simulink model "OFDM_Tx_HW"  (R2020a)
settings: Solver=FixedStepDiscrete  StartTime=0.0  StopTime=inf  RelTol=1e-3
InitFcn:
  | % Set parameters
  | fs = 1e6;
  | 
  | % Load all required variables
  | load('variables/read_addr_data');
  | load('variables/read_addr_cp');
  | load('variables/read_addr_pream');
  | load('variables/read_addr_rx');
  | load('variables/pilot');
  | load('variables/sc_index');
  | load('variables/LTSfreq');
  | load('variables/STSfreq');
  | load('variables/LTSread');
  | load('variables/STSread');
  | 
  | run ./scripts/rfgen;
undefined symbols (not defined in the file or in its folder): CIC_fine_Rx, LTSfreq, LTSread, pilot, read_addr_cp, read_addr_data, read_addr_pream, STSfreq, STSread
libraries: hdlsllib x47, xbsIndex_r4 x30, simulink x19, xrbsSSR_Library x8, dspsigops x5, dspmlti4 x3, lib_ofdmrx x1, lib_rfsignalgenerator x1, dsphdlxfrm x1, dspobslib x1
(part 2 of 2)

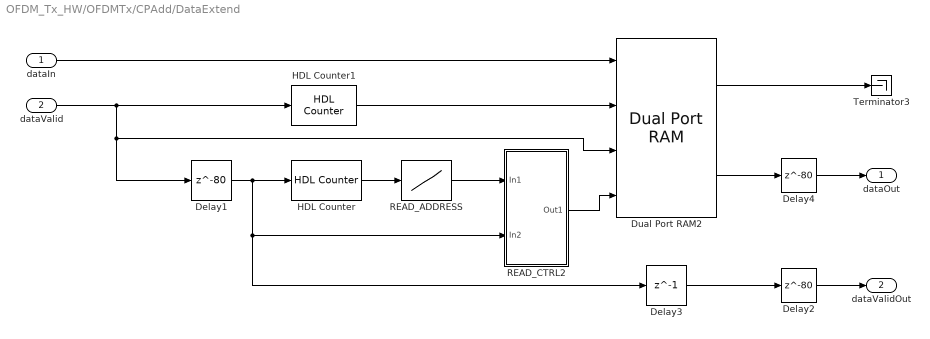
== system OFDM_Tx_HW/OFDMTx/CPAdd/DataExtend ==
  dataIn : Inport
  dataValid : Inport  Port=2
  Delay1 : Delay  DelayLength=80  InitialCondition=0  UseCircularBuffer=on
  Delay2 : Delay  DelayLength=80
  Delay3 : Delay  DelayLength=1  InitialCondition=0  UseCircularBuffer=on
  Delay4 : Delay  DelayLength=80
  Dual Port RAM2 : hdlsllib/HDL RAMs/Dual Port RAM  ram_size=8
      settings: SourceProductBaseCode=SL
  HDL Counter : hdlsllib/Sources/HDL Counter  CountType=Count limited  CountInit=0  CountStep=1  CountMax=159  CountFromType=Initial value  CountFrom=0  CountResetPort=off  CountLoadPort=off  CountEnbPort=on  CountDirPort=off  CountDataType=Unsigned  CountWordLen=8  CountFracLen=0  CountSampTime=1
  HDL Counter1 : hdlsllib/Sources/HDL Counter  CountType=Count limited  CountInit=0  CountStep=1  CountMax=159  CountFromType=Initial value  CountFrom=0  CountResetPort=off  CountLoadPort=off  CountEnbPort=on  CountDirPort=off  CountDataType=Unsigned  CountWordLen=8  CountFracLen=0  CountSampTime=1
  READ_ADDRESS : Lookup_n-D  NumberOfTableDimensions=1  LookupTableObject=''  BreakpointsForDimension1=[0:159]  BreakpointsForDimension1FirstPoint=10  BreakpointsForDimension2FirstPoint=10  BreakpointsForDimension1Spacing=12  BreakpointsForDimension2Spacing=12  IndexSearchMethod=Evenly spaced points  Table=read_addr_cp  TableDataTypeStr=fixdt(0,8,0)  InterpMethod=Flat  DiagnosticForOutOfRangeInput=Error  InternalRulePriority=Speed  OutDataTypeStr=fixdt(0,8,0)  RndMeth=Simplest  InputSameDT=on
  READ_CTRL2 : Subsystem
  Terminator3 : Terminator
  dataOut : Outport  VectorParamsAs1DForOutWhenUnconnected=off
  dataValidOut : Outport  Port=2  VectorParamsAs1DForOutWhenUnconnected=off
  wires:
  Delay4/1 -> dataOut/1
  Delay2/1 -> dataValidOut/1
  Dual Port RAM2/1 -> Terminator3/1
  READ_ADDRESS/1 -> READ_CTRL2/1(In1)
  HDL Counter/1 -> READ_ADDRESS/1
  dataIn/1 -> Dual Port RAM2/1
  HDL Counter1/1 -> Dual Port RAM2/2
  Delay1/1 -> HDL Counter/1, Delay3/1, READ_CTRL2/2(In2)
  Dual Port RAM2/2 -> Delay4/1
  dataValid/1 -> HDL Counter1/1, Dual Port RAM2/3, Delay1/1
  Delay3/1 -> Delay2/1
  READ_CTRL2/1(Out1) -> Dual Port RAM2/4

== system OFDM_Tx_HW/OFDMTx/CPAdd/LTFExtend ==
  data : Inport
  preambVal : Inport  Port=2
  Delay : Delay  DelayLength=160  InitialCondition=0  UseCircularBuffer=on
  Delay12 : Delay  DelayLength=1  InitialCondition=0  UseCircularBuffer=on
  Dual Port RAM : hdlsllib/HDL RAMs/Dual Port RAM  ram_size=8
      settings: SourceProductBaseCode=SL
  HDL Counter2 : hdlsllib/Sources/HDL Counter  CountType=Count limited  CountInit=0  CountStep=1  CountMax=159  CountFromType=Initial value  CountFrom=0  CountResetPort=off  CountLoadPort=off  CountEnbPort=on  CountDirPort=off  CountDataType=Unsigned  CountWordLen=8  CountFracLen=0  CountSampTime=1
  HDL Counter3 : hdlsllib/Sources/HDL Counter  CountType=Count limited  CountInit=0  CountStep=1  CountMax=159  CountFromType=Initial value  CountFrom=0  CountResetPort=off  CountLoadPort=off  CountEnbPort=on  CountDirPort=off  CountDataType=Unsigned  CountWordLen=8  CountFracLen=0  CountSampTime=1
  LTFValidGen : Subsystem
  READ_CTRL : Subsystem
  Terminator1 : Terminator
  readaddr : Lookup_n-D  NumberOfTableDimensions=1  LookupTableObject=''  BreakpointsForDimension1=0:159  BreakpointsForDimension1FirstPoint=10  BreakpointsForDimension2FirstPoint=10  BreakpointsForDimension1Spacing=12  BreakpointsForDimension2Spacing=12  IndexSearchMethod=Evenly spaced points  Table=LTSread  TableDataTypeStr=fixdt(0,8,0)  InterpMethod=Flat  DiagnosticForOutOfRangeInput=Error  InternalRulePriority=Speed  OutDataTypeStr=fixdt(0,8,0)  RndMeth=Simplest  InputSameDT=on
  LTFExtendOut : Outport  VectorParamsAs1DForOutWhenUnconnected=off
  LTFValidOut : Outport  Port=2  VectorParamsAs1DForOutWhenUnconnected=off
  wires:
  readaddr/1 -> READ_CTRL/1(In1)
  READ_CTRL/1(Out1) -> Dual Port RAM/4
  HDL Counter3/1 -> Dual Port RAM/2
  Delay/1 -> READ_CTRL/2(In2), Delay12/1, HDL Counter2/1
  Dual Port RAM/1 -> Terminator1/1
  Delay12/1 -> LTFValidOut/1
  HDL Counter2/1 -> readaddr/1
  data/1 -> Dual Port RAM/1
  Dual Port RAM/2 -> LTFExtendOut/1
  preambVal/1 -> LTFValidGen/1(In1)
  LTFValidGen/1(Out1) -> Dual Port RAM/3, Delay/1, HDL Counter3/1

== system OFDM_Tx_HW/OFDMTx/CPAdd/STFExtend ==
  data : Inport
  preambVal : Inport  Port=2
  Delay : Delay  DelayLength=160  InitialCondition=0  UseCircularBuffer=on
  Delay12 : Delay  DelayLength=1  InitialCondition=0  UseCircularBuffer=on
  Dual Port RAM : hdlsllib/HDL RAMs/Dual Port RAM  ram_size=8
      settings: SourceProductBaseCode=SL
  HDL Counter2 : hdlsllib/Sources/HDL Counter  CountType=Count limited  CountInit=0  CountStep=1  CountMax=159  CountFromType=Initial value  CountFrom=0  CountResetPort=off  CountLoadPort=off  CountEnbPort=on  CountDirPort=off  CountDataType=Unsigned  CountWordLen=8  CountFracLen=0  CountSampTime=1
  HDL Counter3 : hdlsllib/Sources/HDL Counter  CountType=Count limited  CountInit=0  CountStep=1  CountMax=159  CountFromType=Initial value  CountFrom=0  CountResetPort=off  CountLoadPort=off  CountEnbPort=on  CountDirPort=off  CountDataType=Unsigned  CountWordLen=8  CountFracLen=0  CountSampTime=1
  READ_CTRL : Subsystem
  STFValidGen : Subsystem
  Terminator1 : Terminator
  readaddr : Lookup_n-D  NumberOfTableDimensions=1  LookupTableObject=''  BreakpointsForDimension1=0:159  BreakpointsForDimension1FirstPoint=10  BreakpointsForDimension2FirstPoint=10  BreakpointsForDimension1Spacing=12  BreakpointsForDimension2Spacing=12  IndexSearchMethod=Evenly spaced points  Table=STSread  TableDataTypeStr=fixdt(0,8,0)  InterpMethod=Flat  DiagnosticForOutOfRangeInput=Error  InternalRulePriority=Speed  OutDataTypeStr=fixdt(0,8,0)  RndMeth=Simplest  InputSameDT=on
  STFExtendOut : Outport  VectorParamsAs1DForOutWhenUnconnected=off
  STFValidOut : Outport  Port=2  VectorParamsAs1DForOutWhenUnconnected=off
  wires:
  Dual Port RAM/2 -> STFExtendOut/1
  data/1 -> Dual Port RAM/1
  HDL Counter2/1 -> readaddr/1
  Delay12/1 -> STFValidOut/1
  Dual Port RAM/1 -> Terminator1/1
  Delay/1 -> HDL Counter2/1, Delay12/1, READ_CTRL/2(In2)
  HDL Counter3/1 -> Dual Port RAM/2
  READ_CTRL/1(Out1) -> Dual Port RAM/4
  preambVal/1 -> STFValidGen/1(In1)
  readaddr/1 -> READ_CTRL/1(In1)
  STFValidGen/1(Out1) -> HDL Counter3/1, Dual Port RAM/3, Delay/1

== system OFDM_Tx_HW/OFDMTx/ControlSignalGenerator/PreamValidGen ==
  enable : Inport
  Compare To Constant : simulink/Logic and Bit Operations/Compare To Constant  relop===  const=320  OutDataTypeStr=boolean
  HDL Counter : hdlsllib/Sources/HDL Counter  CountType=Count limited  CountInit=0  CountStep=1  CountMax=320  CountFromType=Initial value  CountFrom=0  CountResetPort=on  CountLoadPort=off  CountEnbPort=on  CountDirPort=off  CountDataType=Unsigned  CountWordLen=9  CountFracLen=0  CountSampTime=1
  NOT : Logic  Operator=NOT  IconShape=distinctive  AllPortsSameDT=off  OutDataTypeStr=boolean
  RisingEdge : Subsystem
  Unit Delay Enabled Resettable Synchronous : hdlsllib/Discrete/Unit Delay Enabled Resettable Synchronous  InitialCondition=0.0  SampleTime=-1
      settings: SourceProductBaseCode=SL
  y : Outport  VectorParamsAs1DForOutWhenUnconnected=off
  wires:
  HDL Counter/1 -> Compare To Constant/1
  RisingEdge/1(Out1) -> Unit Delay Enabled Resettable Synchronous/2
  Compare To Constant/1 -> Unit Delay Enabled Resettable Synchronous/3
  enable/1 -> RisingEdge/1(In1), Unit Delay Enabled Resettable Synchronous/1, NOT/1, HDL Counter/2
  Unit Delay Enabled Resettable Synchronous/1 -> y/1
  NOT/1 -> HDL Counter/1

== system OFDM_Tx_HW/OFDMTx/ControlSignalGenerator/dataReadyGen ==
  enb : Inport
  Compare To Constant : simulink/Logic and Bit Operations/Compare To Constant  relop=>  const=31  OutDataTypeStr=boolean
  HDL Counter : hdlsllib/Sources/HDL Counter  CountType=Count limited  CountInit=0  CountStep=1  CountMax=79  CountFromType=Initial value  CountFrom=0  CountResetPort=on  CountLoadPort=off  CountEnbPort=on  CountDirPort=off  CountDataType=Unsigned  CountWordLen=7  CountFracLen=0  CountSampTime=1
  NOT : Logic  Operator=NOT  IconShape=distinctive  AllPortsSameDT=off  OutDataTypeStr=boolean
  y : Outport
  wires:
  HDL Counter/1 -> Compare To Constant/1
  enb/1 -> NOT/1, HDL Counter/2
  NOT/1 -> HDL Counter/1
  Compare To Constant/1 -> y/1

== system OFDM_Tx_HW/OFDMTx/ControlSignalGenerator/dataValidGen ==
  y : Inport
  enable : Inport  Port=2
  AND : Logic  IconShape=distinctive  AllPortsSameDT=off  OutDataTypeStr=boolean
  Delay : Delay  DelayLength=1
  NOT : Logic  Operator=NOT  IconShape=distinctive  AllPortsSameDT=off  OutDataTypeStr=boolean
  valOut : Outport
  wires:
  NOT/1 -> AND/1
  Delay/1 -> AND/2
  AND/1 -> valOut/1
  y/1 -> NOT/1
  enable/1 -> Delay/1

== system OFDM_Tx_HW/OFDMTx/ControlSignalGenerator/pilotValidGen ==
  enb : Inport
  AND : Logic  IconShape=distinctive  AllPortsSameDT=off  OutDataTypeStr=boolean
  Compare To Constant : simulink/Logic and Bit Operations/Compare To Constant  relop=<  const=32  OutDataTypeStr=boolean
  Compare To Constant1 : simulink/Logic and Bit Operations/Compare To Constant  relop=>  const=27  OutDataTypeStr=boolean
  HDL Counter : hdlsllib/Sources/HDL Counter  CountType=Count limited  CountInit=0  CountStep=1  CountMax=79  CountFromType=Initial value  CountFrom=0  CountResetPort=on  CountLoadPort=off  CountEnbPort=on  CountDirPort=off  CountDataType=Unsigned  CountWordLen=7  CountFracLen=0  CountSampTime=1
  NOT : Logic  Operator=NOT  IconShape=distinctive  AllPortsSameDT=off  OutDataTypeStr=boolean
  y : Outport
  wires:
  NOT/1 -> HDL Counter/1
  enb/1 -> HDL Counter/2, NOT/1
  HDL Counter/1 -> Compare To Constant1/1, Compare To Constant/1
  Compare To Constant/1 -> AND/1
  Compare To Constant1/1 -> AND/2
  AND/1 -> y/1

== system OFDM_Tx_HW/OFDMTx/DataGenerator/LTSfreq ==
  preambVal : Inport
  AND : Logic  IconShape=distinctive  AllPortsSameDT=off  OutDataTypeStr=boolean
  AND1 : Logic  IconShape=distinctive  AllPortsSameDT=off  OutDataTypeStr=boolean
  Compare To Constant : simulink/Logic and Bit Operations/Compare To Constant  relop=>=  const=256  OutDataTypeStr=boolean
  Compare To Constant1 : simulink/Logic and Bit Operations/Compare To Constant  relop=<=  const=319  OutDataTypeStr=boolean
  HDL Counter1 : hdlsllib/Sources/HDL Counter  CountType=Count limited  CountInit=0  CountStep=1  CountMax=319  CountFromType=Initial value  CountFrom=0  CountResetPort=on  CountLoadPort=off  CountEnbPort=on  CountDirPort=off  CountDataType=Unsigned  CountWordLen=9  CountFracLen=0  CountSampTime=1
  HDL Counter4 : hdlsllib/Sources/HDL Counter  CountType=Count limited  CountInit=0  CountStep=1  CountMax=63  CountFromType=Initial value  CountFrom=0  CountResetPort=off  CountLoadPort=off  CountEnbPort=on  CountDirPort=off  CountDataType=Unsigned  CountWordLen=6  CountFracLen=0  CountSampTime=1
  LTSFreq : Lookup_n-D  NumberOfTableDimensions=1  LookupTableObject=''  BreakpointsForDimension1=0:63  BreakpointsForDimension1FirstPoint=10  BreakpointsForDimension2FirstPoint=10  BreakpointsForDimension1Spacing=12  BreakpointsForDimension2Spacing=12  IndexSearchMethod=Evenly spaced points  Table=LTSfreq  TableDataTypeStr=fixdt(1,16,14)  InterpMethod=Flat  DiagnosticForOutOfRangeInput=Error  InternalRulePriority=Speed  OutDataTypeStr=fixdt(1,16,14)  RndMeth=Simplest  InputSameDT=on
  NOT : Logic  Operator=NOT  IconShape=distinctive  AllPortsSameDT=off  OutDataTypeStr=boolean
  ltsFreq : Outport  VectorParamsAs1DForOutWhenUnconnected=off
  ltsVal : Outport  Port=2  VectorParamsAs1DForOutWhenUnconnected=off
  wires:
  HDL Counter4/1 -> LTSFreq/1
  Compare To Constant/1 -> AND/1
  HDL Counter1/1 -> Compare To Constant1/1, Compare To Constant/1
  Compare To Constant1/1 -> AND/2
  NOT/1 -> HDL Counter1/1
  AND/1 -> AND1/1
  preambVal/1 -> NOT/1, AND1/2, HDL Counter1/2
  AND1/1 -> ltsVal/1, HDL Counter4/1
  LTSFreq/1 -> ltsFreq/1

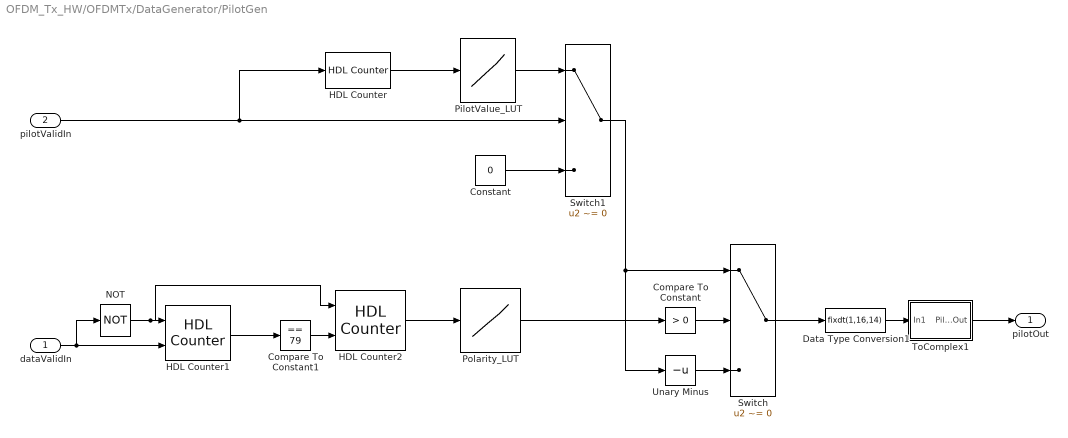
== system OFDM_Tx_HW/OFDMTx/DataGenerator/PilotGen ==
  dataValidIn : Inport
  pilotValidIn : Inport  Port=2
  Compare To Constant : simulink/Logic and Bit Operations/Compare To Constant  relop=>  const=0  OutDataTypeStr=boolean
  Compare To Constant1 : simulink/Logic and Bit Operations/Compare To Constant  relop===  const=79  OutDataTypeStr=boolean
  Constant : Constant  Value=0  OutDataTypeStr=fixdt(1,2,0)  SampleTime=1/fs
  Data Type Conversion1 : DataTypeConversion  OutDataTypeStr=fixdt(1,16,14)
  HDL Counter : hdlsllib/Sources/HDL Counter  CountType=Count limited  CountInit=0  CountStep=1  CountMax=3  CountFromType=Initial value  CountFrom=0  CountResetPort=off  CountLoadPort=off  CountEnbPort=on  CountDirPort=off  CountDataType=Unsigned  CountWordLen=2  CountFracLen=0  CountSampTime=1
  HDL Counter1 : hdlsllib/Sources/HDL Counter  CountType=Count limited  CountInit=0  CountStep=1  CountMax=79  CountFromType=Initial value  CountFrom=0  CountResetPort=on  CountLoadPort=off  CountEnbPort=on  CountDirPort=off  CountDataType=Unsigned  CountWordLen=8  CountFracLen=0  CountSampTime=1
  HDL Counter2 : hdlsllib/Sources/HDL Counter  CountType=Count limited  CountInit=0  CountStep=1  CountMax=126  CountFromType=Initial value  CountFrom=0  CountResetPort=on  CountLoadPort=off  CountEnbPort=on  CountDirPort=off  CountDataType=Unsigned  CountWordLen=7  CountFracLen=0  CountSampTime=1
  NOT : Logic  Operator=NOT  IconShape=distinctive  AllPortsSameDT=off  OutDataTypeStr=boolean
  PilotValue_LUT : Lookup_n-D  NumberOfTableDimensions=1  LookupTableObject=''  BreakpointsForDimension1=[0:3]  BreakpointsForDimension1FirstPoint=10  BreakpointsForDimension2FirstPoint=10  BreakpointsForDimension1Spacing=12  BreakpointsForDimension2Spacing=12  IndexSearchMethod=Evenly spaced points  Table=[1 1 1 -1]  TableDataTypeStr=fixdt(1,2,0)  InterpMethod=Flat  DiagnosticForOutOfRangeInput=Error  InternalRulePriority=Speed  OutDataTypeStr=fixdt(1,2,0)  RndMeth=Simplest  InputSameDT=on
  Polarity_LUT : Lookup_n-D  NumberOfTableDimensions=1  LookupTableObject=''  BreakpointsForDimension1=[0:126]  BreakpointsForDimension1FirstPoint=10  BreakpointsForDimension2FirstPoint=10  BreakpointsForDimension1Spacing=12  BreakpointsForDimension2Spacing=12  IndexSearchMethod=Evenly spaced points  Table=pilot  TableDataTypeStr=fixdt(1,2,0)  InterpMethod=Flat  DiagnosticForOutOfRangeInput=Error  InternalRulePriority=Speed  OutDataTypeStr=fixdt(1,2,0)  RndMeth=Simplest  InputSameDT=on
  Switch : Switch  Criteria=u2 ~= 0
  Switch1 : Switch  Criteria=u2 ~= 0
  ToComplex1 : Subsystem
  Unary Minus : UnaryMinus
  pilotOut : Outport  VectorParamsAs1DForOutWhenUnconnected=off
  wires:
  HDL Counter/1 -> PilotValue_LUT/1
  Data Type Conversion1/1 -> ToComplex1/1(In1)
  dataValidIn/1 -> HDL Counter1/2, NOT/1
  HDL Counter1/1 -> Compare To Constant1/1
  NOT/1 -> HDL Counter2/1, HDL Counter1/1
  Compare To Constant1/1 -> HDL Counter2/2
  HDL Counter2/1 -> Polarity_LUT/1
  ToComplex1/1(PilotOut) -> pilotOut/1
  pilotValidIn/1 -> HDL Counter/1, Switch1/2
  Polarity_LUT/1 -> Compare To Constant/1
  Compare To Constant/1 -> Switch/2
  Unary Minus/1 -> Switch/3
  Switch/1 -> Data Type Conversion1/1
  PilotValue_LUT/1 -> Switch1/1
  Switch1/1 -> Unary Minus/1, Switch/1
  Constant/1 -> Switch1/3

== system OFDM_Tx_HW/OFDMTx/DataGenerator/STSFreq ==
  preamVal : Inport
  AND : Logic  IconShape=distinctive  AllPortsSameDT=off  OutDataTypeStr=boolean
  AND1 : Logic  IconShape=distinctive  AllPortsSameDT=off  OutDataTypeStr=boolean
  Compare To Constant : simulink/Logic and Bit Operations/Compare To Constant  relop=>=  const=96  OutDataTypeStr=boolean
  Compare To Constant1 : simulink/Logic and Bit Operations/Compare To Constant  relop=<=  const=159  OutDataTypeStr=boolean
  HDL Counter : hdlsllib/Sources/HDL Counter  CountType=Count limited  CountInit=0  CountStep=1  CountMax=63  CountFromType=Initial value  CountFrom=0  CountResetPort=off  CountLoadPort=off  CountEnbPort=on  CountDirPort=off  CountDataType=Unsigned  CountWordLen=6  CountFracLen=0  CountSampTime=1
  HDL Counter1 : hdlsllib/Sources/HDL Counter  CountType=Count limited  CountInit=0  CountStep=1  CountMax=319  CountFromType=Initial value  CountFrom=0  CountResetPort=on  CountLoadPort=off  CountEnbPort=on  CountDirPort=off  CountDataType=Unsigned  CountWordLen=9  CountFracLen=0  CountSampTime=1
  NOT : Logic  Operator=NOT  IconShape=distinctive  AllPortsSameDT=off  OutDataTypeStr=boolean
  STSFreq : Lookup_n-D  NumberOfTableDimensions=1  LookupTableObject=''  BreakpointsForDimension1=[0:63]  BreakpointsForDimension1FirstPoint=10  BreakpointsForDimension2FirstPoint=10  BreakpointsForDimension1Spacing=12  BreakpointsForDimension2Spacing=12  IndexSearchMethod=Evenly spaced points  Table=STSfreq  TableDataTypeStr=fixdt(1,16,14)  InterpMethod=Flat  DiagnosticForOutOfRangeInput=Error  InternalRulePriority=Speed  OutDataTypeStr=fixdt(1,16,14)  RndMeth=Simplest  InputSameDT=on
  stsFreq : Outport  VectorParamsAs1DForOutWhenUnconnected=off
  stsVal : Outport  Port=2  VectorParamsAs1DForOutWhenUnconnected=off
  wires:
  HDL Counter/1 -> STSFreq/1
  AND/1 -> AND1/1
  HDL Counter1/1 -> Compare To Constant1/1, Compare To Constant/1
  NOT/1 -> HDL Counter1/1
  Compare To Constant/1 -> AND/1
  Compare To Constant1/1 -> AND/2
  preamVal/1 -> NOT/1, AND1/2, HDL Counter1/2
  AND1/1 -> stsVal/1, HDL Counter/1
  STSFreq/1 -> stsFreq/1

== system OFDM_Tx_HW/OFDMTx/IFFT/IFFTValid ==
  preambleValid : Inport
  dataValid : Inport  Port=2
  Switch : Switch  Criteria=u2 ~= 0
  dataIFFTValid : Subsystem
  preambIFFTValid : Subsystem
  ifftValid : Outport  VectorParamsAs1DForOutWhenUnconnected=off
  wires:
  preambleValid/1 -> Switch/2, preambIFFTValid/1(preambValid)
  preambIFFTValid/1(preambIFFTValidOut) -> Switch/1
  dataValid/1 -> dataIFFTValid/1(dataValidIn)
  dataIFFTValid/1(dataIFFTValidOut) -> Switch/3
  Switch/1 -> ifftValid/1

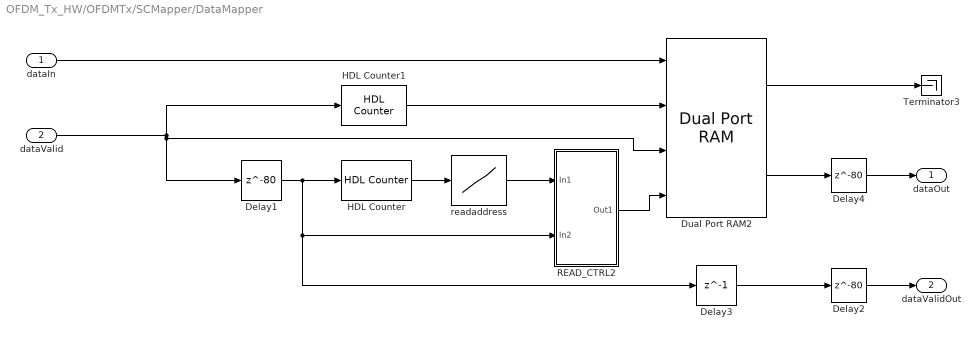
== system OFDM_Tx_HW/OFDMTx/SCMapper/DataMapper ==
  dataIn : Inport
  dataValid : Inport  Port=2
  Delay1 : Delay  DelayLength=80  InitialCondition=0  UseCircularBuffer=on
  Delay2 : Delay  DelayLength=80
  Delay3 : Delay  DelayLength=1  InitialCondition=0  UseCircularBuffer=on
  Delay4 : Delay  DelayLength=80
  Dual Port RAM2 : hdlsllib/HDL RAMs/Dual Port RAM  ram_size=8
      settings: SourceProductBaseCode=SL
  HDL Counter : hdlsllib/Sources/HDL Counter  CountType=Count limited  CountInit=0  CountStep=1  CountMax=159  CountFromType=Initial value  CountFrom=0  CountResetPort=off  CountLoadPort=off  CountEnbPort=on  CountDirPort=off  CountDataType=Unsigned  CountWordLen=8  CountFracLen=0  CountSampTime=1
  HDL Counter1 : hdlsllib/Sources/HDL Counter  CountType=Count limited  CountInit=0  CountStep=1  CountMax=159  CountFromType=Initial value  CountFrom=0  CountResetPort=off  CountLoadPort=off  CountEnbPort=on  CountDirPort=off  CountDataType=Unsigned  CountWordLen=8  CountFracLen=0  CountSampTime=1
  READ_CTRL2 : Subsystem
  Terminator3 : Terminator
  readaddress : Lookup_n-D  NumberOfTableDimensions=1  LookupTableObject=''  BreakpointsForDimension1=[0:159]  BreakpointsForDimension1FirstPoint=10  BreakpointsForDimension2FirstPoint=10  BreakpointsForDimension1Spacing=12  BreakpointsForDimension2Spacing=12  IndexSearchMethod=Evenly spaced points  Table=read_addr_data  TableDataTypeStr=fixdt(0,8,0)  InterpMethod=Flat  DiagnosticForOutOfRangeInput=Error  InternalRulePriority=Speed  OutDataTypeStr=fixdt(0,8,0)  RndMeth=Simplest  InputSameDT=on
  dataOut : Outport  VectorParamsAs1DForOutWhenUnconnected=off
  dataValidOut : Outport  Port=2  VectorParamsAs1DForOutWhenUnconnected=off
  wires:
  READ_CTRL2/1(Out1) -> Dual Port RAM2/4
  Delay3/1 -> Delay2/1
  dataValid/1 -> HDL Counter1/1, Delay1/1, Dual Port RAM2/3
  Dual Port RAM2/2 -> Delay4/1
  Delay1/1 -> READ_CTRL2/2(In2), Delay3/1, HDL Counter/1
  HDL Counter1/1 -> Dual Port RAM2/2
  dataIn/1 -> Dual Port RAM2/1
  HDL Counter/1 -> readaddress/1
  readaddress/1 -> READ_CTRL2/1(In1)
  Dual Port RAM2/1 -> Terminator3/1
  Delay2/1 -> dataValidOut/1
  Delay4/1 -> dataOut/1

== system OFDM_Tx_HW/OFDMTx/SCMapper/PremableMapper ==
  data : Inport
  preambVal : Inport  Port=2
  Delay : Delay  DelayLength=160  InitialCondition=0  UseCircularBuffer=on
  Delay12 : Delay  DelayLength=1  InitialCondition=0  UseCircularBuffer=on
  Dual Port RAM : hdlsllib/HDL RAMs/Dual Port RAM  ram_size=9
      settings: SourceProductBaseCode=SL
  HDL Counter2 : hdlsllib/Sources/HDL Counter  CountType=Count limited  CountInit=0  CountStep=1  CountMax=319  CountFromType=Initial value  CountFrom=0  CountResetPort=off  CountLoadPort=off  CountEnbPort=on  CountDirPort=off  CountDataType=Unsigned  CountWordLen=9  CountFracLen=0  CountSampTime=1
  HDL Counter3 : hdlsllib/Sources/HDL Counter  CountType=Count limited  CountInit=0  CountStep=1  CountMax=319  CountFromType=Initial value  CountFrom=0  CountResetPort=off  CountLoadPort=off  CountEnbPort=on  CountDirPort=off  CountDataType=Unsigned  CountWordLen=9  CountFracLen=0  CountSampTime=1
  READ_CTRL : Subsystem
  Terminator1 : Terminator
  readaddr : Lookup_n-D  NumberOfTableDimensions=1  LookupTableObject=''  BreakpointsForDimension1=0:319  BreakpointsForDimension1FirstPoint=10  BreakpointsForDimension2FirstPoint=10  BreakpointsForDimension1Spacing=12  BreakpointsForDimension2Spacing=12  IndexSearchMethod=Evenly spaced points  Table=read_addr_pream  TableDataTypeStr=fixdt(0,9,0)  InterpMethod=Flat  DiagnosticForOutOfRangeInput=Error  InternalRulePriority=Speed  OutDataTypeStr=fixdt(0,9,0)  RndMeth=Simplest  InputSameDT=on
  preambleShiftOut : Outport  VectorParamsAs1DForOutWhenUnconnected=off
  preambValOut : Outport  Port=2  VectorParamsAs1DForOutWhenUnconnected=off
  wires:
  readaddr/1 -> READ_CTRL/1(In1)
  preambVal/1 -> Delay/1, Dual Port RAM/3, HDL Counter3/1
  READ_CTRL/1(Out1) -> Dual Port RAM/4
  HDL Counter3/1 -> Dual Port RAM/2
  Delay/1 -> READ_CTRL/2(In2), Delay12/1, HDL Counter2/1
  Dual Port RAM/1 -> Terminator1/1
  Delay12/1 -> preambValOut/1
  HDL Counter2/1 -> readaddr/1
  data/1 -> Dual Port RAM/1
  Dual Port RAM/2 -> preambleShiftOut/1

== system OFDM_Tx_HW/OFDMTx/CPAdd/DataExtend/READ_CTRL2 ==
  In1 : Inport
  In2 : Inport  Port=2
  Constant : Constant  Value=0  OutDataTypeStr=fixdt(0,8,0)  SampleTime=1/fs
  Switch : Switch  Criteria=u2 ~= 0
  Out1 : Outport  VectorParamsAs1DForOutWhenUnconnected=off
  wires:
  Constant/1 -> Switch/3
  In2/1 -> Switch/2
  In1/1 -> Switch/1
  Switch/1 -> Out1/1

== system OFDM_Tx_HW/OFDMTx/CPAdd/LTFExtend/LTFValidGen ==
  In1 : Inport
  AND : Logic  IconShape=distinctive  AllPortsSameDT=off  OutDataTypeStr=boolean
  AND1 : Logic  IconShape=distinctive  AllPortsSameDT=off  OutDataTypeStr=boolean
  Compare To Constant : simulink/Logic and Bit Operations/Compare To Constant  relop=>=  const=160  OutDataTypeStr=boolean
  Compare To Constant1 : simulink/Logic and Bit Operations/Compare To Constant  relop=<=  const=319  OutDataTypeStr=boolean
  HDL Counter : hdlsllib/Sources/HDL Counter  CountType=Count limited  CountInit=0  CountStep=1  CountMax=319  CountFromType=Initial value  CountFrom=0  CountResetPort=on  CountLoadPort=off  CountEnbPort=on  CountDirPort=off  CountDataType=Unsigned  CountWordLen=9  CountFracLen=0  CountSampTime=1
  NOT : Logic  Operator=NOT  IconShape=distinctive  AllPortsSameDT=off  OutDataTypeStr=boolean
  Out1 : Outport  VectorParamsAs1DForOutWhenUnconnected=off
  wires:
  Compare To Constant/1 -> AND/1
  In1/1 -> NOT/1, AND1/2, HDL Counter/2
  HDL Counter/1 -> Compare To Constant1/1, Compare To Constant/1
  Compare To Constant1/1 -> AND/2
  AND1/1 -> Out1/1
  AND/1 -> AND1/1
  NOT/1 -> HDL Counter/1

== system OFDM_Tx_HW/OFDMTx/CPAdd/LTFExtend/READ_CTRL ==
  In1 : Inport
  In2 : Inport  Port=2
  Constant : Constant  Value=0  OutDataTypeStr=fixdt(0,8,0)  SampleTime=1/fs
  Switch : Switch  Criteria=u2 ~= 0
  Out1 : Outport  VectorParamsAs1DForOutWhenUnconnected=off
  wires:
  Switch/1 -> Out1/1
  In1/1 -> Switch/1
  In2/1 -> Switch/2
  Constant/1 -> Switch/3

== system OFDM_Tx_HW/OFDMTx/CPAdd/STFExtend/READ_CTRL ==
  In1 : Inport
  In2 : Inport  Port=2
  Constant : Constant  Value=0  OutDataTypeStr=fixdt(0,8,0)  SampleTime=1/fs
  Switch : Switch  Criteria=u2 ~= 0
  Out1 : Outport  VectorParamsAs1DForOutWhenUnconnected=off
  wires:
  Constant/1 -> Switch/3
  In2/1 -> Switch/2
  In1/1 -> Switch/1
  Switch/1 -> Out1/1

== system OFDM_Tx_HW/OFDMTx/CPAdd/STFExtend/STFValidGen ==
  In1 : Inport
  AND : Logic  IconShape=distinctive  AllPortsSameDT=off  OutDataTypeStr=boolean
  AND1 : Logic  IconShape=distinctive  AllPortsSameDT=off  OutDataTypeStr=boolean
  Compare To Constant : simulink/Logic and Bit Operations/Compare To Constant  relop=>=  const=0  OutDataTypeStr=boolean
  Compare To Constant1 : simulink/Logic and Bit Operations/Compare To Constant  relop=<=  const=159  OutDataTypeStr=boolean
  HDL Counter : hdlsllib/Sources/HDL Counter  CountType=Count limited  CountInit=0  CountStep=1  CountMax=319  CountFromType=Initial value  CountFrom=0  CountResetPort=on  CountLoadPort=off  CountEnbPort=on  CountDirPort=off  CountDataType=Unsigned  CountWordLen=9  CountFracLen=0  CountSampTime=1
  NOT : Logic  Operator=NOT  IconShape=distinctive  AllPortsSameDT=off  OutDataTypeStr=boolean
  Out1 : Outport  VectorParamsAs1DForOutWhenUnconnected=off
  wires:
  Compare To Constant/1 -> AND/1
  In1/1 -> NOT/1, AND1/2, HDL Counter/2
  HDL Counter/1 -> Compare To Constant1/1, Compare To Constant/1
  Compare To Constant1/1 -> AND/2
  AND1/1 -> Out1/1
  AND/1 -> AND1/1
  NOT/1 -> HDL Counter/1

== system OFDM_Tx_HW/OFDMTx/ControlSignalGenerator/PreamValidGen/RisingEdge ==
  In1 : Inport
  Delay : Delay  DelayLength=1
  Relational Operator : RelationalOperator  Operator=>  OutDataTypeStr=boolean  RndMeth=Nearest
  Out1 : Outport
  wires:
  Relational Operator/1 -> Out1/1
  Delay/1 -> Relational Operator/2
  In1/1 -> Delay/1, Relational Operator/1

== system OFDM_Tx_HW/OFDMTx/DataGenerator/PilotGen/ToComplex1 ==
  In1 : Inport
  Constant1 : Constant  Value=0  OutDataTypeStr=fixdt(1,16,14)  SampleTime=1/fs
  Real-Imag to Complex : RealImagToComplex
  PilotOut : Outport  VectorParamsAs1DForOutWhenUnconnected=off
  wires:
  Constant1/1 -> Real-Imag to Complex/2
  In1/1 -> Real-Imag to Complex/1
  Real-Imag to Complex/1 -> PilotOut/1

== system OFDM_Tx_HW/OFDMTx/IFFT/IFFTValid/dataIFFTValid ==
  dataValidIn : Inport
  Compare To Constant : simulink/Logic and Bit Operations/Compare To Constant  relop=>=  const=17  OutDataTypeStr=boolean
  Logical Operator : Logic  Operator=NOT  IconShape=distinctive  AllPortsSameDT=off  OutDataTypeStr=boolean
  SAMPLE_COUNTER : hdlsllib/Sources/HDL Counter  CountType=Count limited  CountInit=1  CountStep=1  CountMax=80  CountFromType=Initial value  CountFrom=1  CountResetPort=on  CountLoadPort=off  CountEnbPort=on  CountDirPort=off  CountDataType=Unsigned  CountWordLen=7  CountFracLen=0  CountSampTime=1
  dataIFFTValidOut : Outport  VectorParamsAs1DForOutWhenUnconnected=off
  wires:
  dataValidIn/1 -> SAMPLE_COUNTER/2, Logical Operator/1
  Compare To Constant/1 -> dataIFFTValidOut/1
  Logical Operator/1 -> SAMPLE_COUNTER/1
  SAMPLE_COUNTER/1 -> Compare To Constant/1

== system OFDM_Tx_HW/OFDMTx/IFFT/IFFTValid/preambIFFTValid ==
  preambValid : Inport
  AND{,1..3} (4 alike) : Logic  IconShape=distinctive  AllPortsSameDT=off  OutDataTypeStr=boolean
  Compare To Constant1 : simulink/Logic and Bit Operations/Compare To Constant  relop=>=  const=96  OutDataTypeStr=boolean
  Compare To Constant2 : simulink/Logic and Bit Operations/Compare To Constant  relop=<=  const=159  OutDataTypeStr=boolean
  Compare To Constant3 : simulink/Logic and Bit Operations/Compare To Constant  relop=>=  const=256  OutDataTypeStr=boolean
  Compare To Constant4 : simulink/Logic and Bit Operations/Compare To Constant  relop=<=  const=319  OutDataTypeStr=boolean
  HDL Counter1 : hdlsllib/Sources/HDL Counter  CountType=Count limited  CountInit=0  CountStep=1  CountMax=319  CountFromType=Initial value  CountFrom=0  CountResetPort=on  CountLoadPort=off  CountEnbPort=on  CountDirPort=off  CountDataType=Unsigned  CountWordLen=9  CountFracLen=0  CountSampTime=1
  NOT : Logic  Operator=NOT  IconShape=distinctive  AllPortsSameDT=off  OutDataTypeStr=boolean
  OR : Logic  Operator=OR  IconShape=distinctive  AllPortsSameDT=off  OutDataTypeStr=boolean
  preambIFFTValidOut : Outport  VectorParamsAs1DForOutWhenUnconnected=off
  wires:
  AND/1 -> AND1/1
  AND2/1 -> AND3/1
  HDL Counter1/1 -> Compare To Constant4/1, Compare To Constant3/1, Compare To Constant2/1, Compare To Constant1/1
  OR/1 -> preambIFFTValidOut/1
  preambValid/1 -> HDL Counter1/2, AND3/2, AND1/2, NOT/1
  Compare To Constant1/1 -> AND/1
  Compare To Constant4/1 -> AND2/2
  AND1/1 -> OR/1
  AND3/1 -> OR/2
  Compare To Constant2/1 -> AND/2
  NOT/1 -> HDL Counter1/1
  Compare To Constant3/1 -> AND2/1

== system OFDM_Tx_HW/OFDMTx/SCMapper/DataMapper/READ_CTRL2 ==
  In1 : Inport
  In2 : Inport  Port=2
  Constant : Constant  Value=0  OutDataTypeStr=fixdt(0,8,0)  SampleTime=1/fs
  Switch : Switch  Criteria=u2 ~= 0
  Out1 : Outport  VectorParamsAs1DForOutWhenUnconnected=off
  wires:
  Switch/1 -> Out1/1
  In1/1 -> Switch/1
  In2/1 -> Switch/2
  Constant/1 -> Switch/3

== system OFDM_Tx_HW/OFDMTx/SCMapper/PremableMapper/READ_CTRL ==
  In1 : Inport
  In2 : Inport  Port=2
  Constant : Constant  Value=0  OutDataTypeStr=fixdt(0,8,0)  SampleTime=1/fs
  Switch : Switch  Criteria=u2 ~= 0
  Out1 : Outport  VectorParamsAs1DForOutWhenUnconnected=off
  wires:
  Switch/1 -> Out1/1
  In1/1 -> Switch/1
  In2/1 -> Switch/2
  Constant/1 -> Switch/3

== matlab function OFDM_Tx_HW/OFDMTx/DataGenerator/Data Multiplexer ==
  data: symbols input; dataready input; data output; pilots input; pval input; sts input; stsval input; lts input; ltsval input
function data  = dataMux(symbols,dataready,pilots,pval,sts,stsval,lts,ltsval)
% Data multiplexer 
if (pval == true)
    data = pilots; 
elseif (stsval == true)
    data = sts; 
elseif (ltsval == true)
    data = lts; 
elseif (dataready == true) 
    data = symbols;
else 
    data = fi(complex(0),1,16,14);
end

== matlab function OFDM_Tx_HW/OFDMTx/CPAdd/Mux2 ==
  data: sts input; stsval input; lts input; ltsval input; dataOut output; data input; dataval input
function dataOut = mux(sts,stsval,lts,ltsval,data,dataval)

if (stsval == true)
    dataOut = sts; 
elseif (ltsval == true)
    dataOut = lts; 
elseif (dataval == true) 
    dataOut = data; 
else 
    dataOut = fi(complex(0),1,16,14);
end

== matlab function OFDM_Tx_HW/OFDMTx/SCMapper/Mux2 ==
  data: preamb input; preambVal input; dataOut output; data input; dataVal input
function dataOut = mux(preamb,preambVal,data,dataVal)

if (preambVal == true)
    dataOut = preamb; 
elseif (dataVal == true)
    dataOut = data; 
else 
    dataOut = fi(complex(0),1,16,14);
end
